simulink model "inv_cin"  (R2020b)
settings: Solver=VariableStepAuto  StartTime=1  StopTime=39  RelTol=1e-3
libraries: simulink x2
settings Model: PacingRate=3  Creator=beatr  LastModifiedBy=Stefano
settings SolverCC: ZeroCrossAlgorithm=Adaptive
settings DebuggingCC: IgnoredZcDiagnostic=none

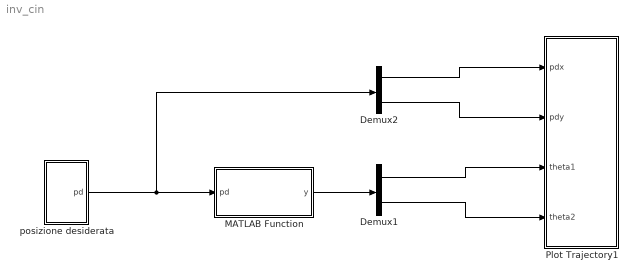
== system inv_cin ==
  Demux1 : Demux  Outputs=2
  Demux2 : Demux  Outputs=2
  MATLAB Function : MATLAB Function  TreatAsAtomicUnit=on
  Plot Trajectory1 : MATLAB Function  TreatAsAtomicUnit=on  SystemSampleTime=1
  posizione desiderata : Subsystem
  wires:
  Demux2/2 -> Plot Trajectory1/2(pdy)
  Demux2/1 -> Plot Trajectory1/1(pdx)
  MATLAB Function/1(y) -> Demux1/1
  Demux1/1 -> Plot Trajectory1/3(theta1)
  Demux1/2 -> Plot Trajectory1/4(theta2)
  posizione desiderata/1(pd) -> MATLAB Function/1(pd), Demux2/1

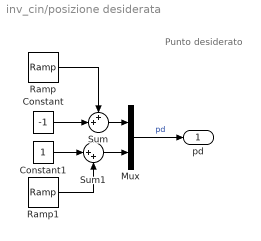
== system inv_cin/posizione desiderata ==
  note: Punto desiderato
  Constant : Constant  Value=-1
  Constant1 : Constant
  Mux : Mux  Inputs=2
  Ramp : simulink/Sources/Ramp  slope=1/10  start=10  InitialOutput=0
  Ramp1 : simulink/Sources/Ramp  slope=-0.5/10  start=10  InitialOutput=0
  Sum : Sum  Inputs=++|
  Sum1 : Sum  Inputs=|++
  pd : Outport
  wires:
  Constant/1 -> Sum/2
  Mux/1 -> pd/1  "pd"
  Sum/1 -> Mux/1
  Ramp/1 -> Sum/1
  Constant1/1 -> Sum1/1
  Sum1/1 -> Mux/2
  Ramp1/1 -> Sum1/2

== matlab function inv_cin/Plot Trajectory1 ==
  settings: updateMethod=DISCRETE
  data: pdx input; pdy input; theta1 input; theta2 input
function PlotTraiettoria(pdx,pdy,theta1,theta2)

eml.extrinsic('findobj','get','set','figure','clf',...
              'hold','delete','plot','axis','grid',...
              'hggroup','quiver','drawnow','num2str');
          
persistent target;
persistent chain;
persistent velocity;
persistent chain2;
persistent i;
persistent deleted_fig;

          
pex=[0;cos(theta1);cos(theta1)+cos(theta1+theta2)];

pey=[0;sin(theta1);sin(theta1)+sin(theta1+theta2)];


foundFig=findobj('Tag','trajScope');

if isempty(deleted_fig)
    deleted_fig=1;
    % La prima volta cancello la figura
    if ~isempty(foundFig)
        delete(foundFig)   
    end      
end


foundFig=findobj('Tag','trajScope');


if isempty(foundFig)
    fig=figure('Color','white');
    clf(fig);
    set(fig,'Name','Trajectory');
    set(fig,'DoubleBuffer','on','Tag','trajScope');
    set(fig,'Renderer','painters');
    hold('on');
    hax=get(fig,'CurrentAxes');
    set(hax,'DrawMode','fast','Box','off');    
    
    %target=plot(hax,pdx,pdy,'bo','MarkerFaceColor','b');

    chain=hggroup;
    h1=plot(hax,pex,pey,'r','LineWidth',3);
    h2=plot(hax,pex(1),pey(1),'ro','MarkerFaceColor','r');
    h3=plot(hax,pex(2),pey(2),'ro','MarkerFaceColor','r');
    h4=plot(hax,pex(3),pey(3),'ro','MarkerFaceColor','r');
    set(h1,'Parent',chain);
    set(h2,'Parent',chain);
    set(h3,'Parent',chain);
    set(h4,'Parent',chain);
    
    % draw the desired point
    target=plot(hax,pdx,pdy,'bo','MarkerFaceColor','b');

    
    axis([-2.3 2.3 -2.3 2.3]);
    axis('equal');
    grid('on');
else
    hax=get(foundFig,'CurrentAxes');
end


if ~isempty(chain)
    delete(chain);
end
if ~isempty(target)
    %delete(target);
end


% draw the desired point
target=plot(hax,pdx,pdy,'bo','MarkerFaceColor','b');

% draw the link
chain=hggroup;
h1=plot(hax,pex,pey,'r','LineWidth',3);
h2=plot(hax,pex(1),pey(1),'ro','MarkerFaceColor','r');
h3=plot(hax,pex(2),pey(2),'ro','MarkerFaceColor','r');
h4=plot(hax,pex(3),pey(3),'ro','MarkerFaceColor','r');
set(h1,'Parent',chain);
set(h2,'Parent',chain);
set(h3,'Parent',chain);
set(h4,'Parent',chain);


% draw the end-effector velocity in the cartesian space
%velocity=quiver(hax,pex(end),pey(end),vex,vey,'Color','green','LineWidth',2);

title([num2str(theta1) ' ; ' num2str(theta2)])

axis([-3 3 -3 3])
drawnow;

== matlab function inv_cin/MATLAB Function ==
  data: pd input; y output
function y = cinematica_inversa(pd)

a1=1;
a2=1;

y=zeros(2,1);

c2=(pd(1)^2+pd(2)^2-a1^2-a2^2)/(2*a1*a2);

y(2)=acos(c2);


alpha= atan2(pd(2),pd(1));

a=(pd(1)^2+pd(2)^2+a1^2-a2^2)/(2*a1*sqrt(pd(1)^2+pd(2)^2));

beta=acos(a);

y(1)=alpha-beta;
